simulink model "main_22a"  (R2022a)
settings: Solver=ode4  StartTime=0.0  StopTime=1  FixedStep=deltat  RelTol=1e-3
model workspace (MAT data in the model file):
  Dutyfactor = Simulink.Parameter
  Dutyfactor.Value = 0.25
  Dutyfactor.DataType = 'double'
  Dutyfactor.Complexity = 'real'
  Dutyfactor.Dimensions = [1 1]
  LenghtOfBot = Simulink.Parameter
  LenghtOfBot.Value = 0.5
  LenghtOfBot.DataType = 'double'
  LenghtOfBot.Complexity = 'real'
  LenghtOfBot.Dimensions = [1 1]
  MomentOfInertia = Simulink.Parameter
  MomentOfInertia.Value = [0.41  0  0; 0  2.1  0; 0  0  2.1]
  MomentOfInertia.DataType = 'double'
  MomentOfInertia.Complexity = 'real'
  MomentOfInertia.Dimensions = [3 3]
  Q = Simulink.Parameter
  Q.Value = [100  0  0  0  0  0  0  0  0  0  0  0; 0  100  0  0  0  0  0  0  0  0  0  0; 0  0  100  0  0  0  0  0  0  0  0  0; 0  0  0  100  0  0  0  0  0  0  0  0; 0  0  0  0  100  0  0  0  0  0  0  0; 0  0  0  0  0  100  0  0  0  0  0  0; 0  0  0  0  0  0  100  0  0  0  0  0; 0  0  0  0  0  0  0  100  0  0  0  0; 0  0  0  0  0  0  0  0  100  0  0  0; 0  0  0  0  0  0  0  0  0  100  0  0; 0  0  0  0  0  0  0  0  0  0  100  0; 0  0  0  0  0  0  0  0  0  0  0  100]
  Q.DataType = 'double'
  Q.Complexity = 'real'
  Q.Dimensions = [12 12]
  R = Simulink.Parameter
  R.Value = [1e-05  0  0  0  0  0  0  0  0  0  0  0; 0  1e-05  0  0  0  0  0  0  0  0  0  0; 0  0  1e-05  0  0  0  0  0  0  0  0  0; 0  0  0  1e-05  0  0  0  0  0  0  0  0; 0  0  0  0  1e-05  0  0  0  0  0  0  0; 0  0  0  0  0  1e-05  0  0  0  0  0  0; 0  0  0  0  0  0  1e-05  0  0  0  0  0; 0  0  0  0  0  0  0  1e-05  0  0  0  0; 0  0  0  0  0  0  0  0  1e-05  0  0  0; 0  0  0  0  0  0  0  0  0  1e-05  0  0; 0  0  0  0  0  0  0  0  0  0  1e-05  0; 0  0  0  0  0  0  0  0  0  0  0  1e-05]
  R.DataType = 'double'
  R.Complexity = 'real'
  R.Dimensions = [12 12]
  RelativePhase = Simulink.Parameter
  RelativePhase.Value = [0; 0.5; 0.75; 0.25]
  RelativePhase.DataType = 'double'
  RelativePhase.Complexity = 'real'
  RelativePhase.Dimensions = [4 1]
  WidthOfBot = Simulink.Parameter
  WidthOfBot.Value = 0.3
  WidthOfBot.DataType = 'double'
  WidthOfBot.Complexity = 'real'
  WidthOfBot.Dimensions = [1 1]
  cycleTime = Simulink.Parameter
  cycleTime.Value = 1
  cycleTime.DataType = 'double'
  cycleTime.Complexity = 'real'
  cycleTime.Dimensions = [1 1]
  deltat = Simulink.Parameter
  deltat.Value = 0.05
  deltat.DataType = 'double'
  deltat.Complexity = 'real'
  deltat.Dimensions = [1 1]
  fmax = Simulink.Parameter
  fmax.Value = 666
  fmax.DataType = 'double'
  fmax.Complexity = 'real'
  fmax.Dimensions = [1 1]
  fmin = Simulink.Parameter
  fmin.Value = 10
  fmin.DataType = 'double'
  fmin.Complexity = 'real'
  fmin.Dimensions = [1 1]
  gravity = Simulink.Parameter
  gravity.Value = [0; 0; -9.8]
  gravity.DataType = 'double'
  gravity.Complexity = 'real'
  gravity.Dimensions = [3 1]
  mass = Simulink.Parameter
  mass.Value = 43
  mass.DataType = 'double'
  mass.Complexity = 'real'
  mass.Dimensions = [1 1]
  mu = Simulink.Parameter
  mu.Value = 0.6
  mu.DataType = 'double'
  mu.Complexity = 'real'
  mu.Dimensions = [1 1]
  nominal_height = Simulink.Parameter
  nominal_height.Value = 0.2
  nominal_height.DataType = 'double'
  nominal_height.Complexity = 'real'
  nominal_height.Dimensions = [1 1]
  number_of_timeStepsMPC = Simulink.Parameter
  number_of_timeStepsMPC.Value = 1
  number_of_timeStepsMPC.DataType = 'int8'
  number_of_timeStepsMPC.Complexity = 'real'
  number_of_timeStepsMPC.Dimensions = [1 1]
values from neighbouring files (symbols this model uses):
  fmax = 660    [main24.m]
  fmin = 10    [main24.m]
  mu = 0.6    [main24.m]
  Q = zeros(13*n_steps,13*n_steps)    [Active_set_QP.m]    (also in main24.m = eye(12,12)*100)
  R = zeros(size(Bqp,2),size(Bqp,2))    [Active_set_QP.m]    (also in Aqp_Bqp.m = [0 -r(3) r(2);r(3) 0 -r(1);-r(2) r(1) 0]; main24.m = eye(12,12)*10^-2)
settings Model: Creator=user  LastModifiedBy=user
settings ModelReferenceCC: EnableRefExpFcnMdlSchedulingChecks=off
settings RTWCC: Description=Generic Real-Time Target

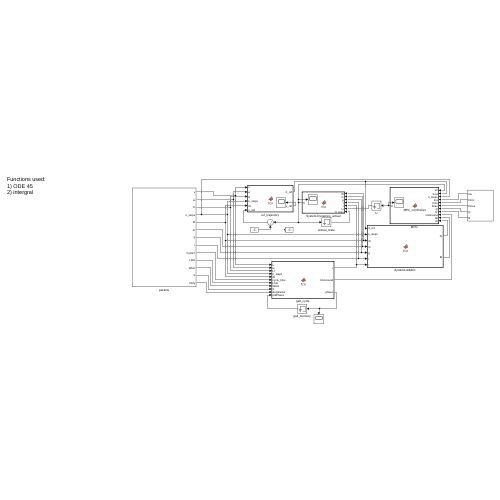
[thumbnail: Simulink's stored preview of the top-level diagram]
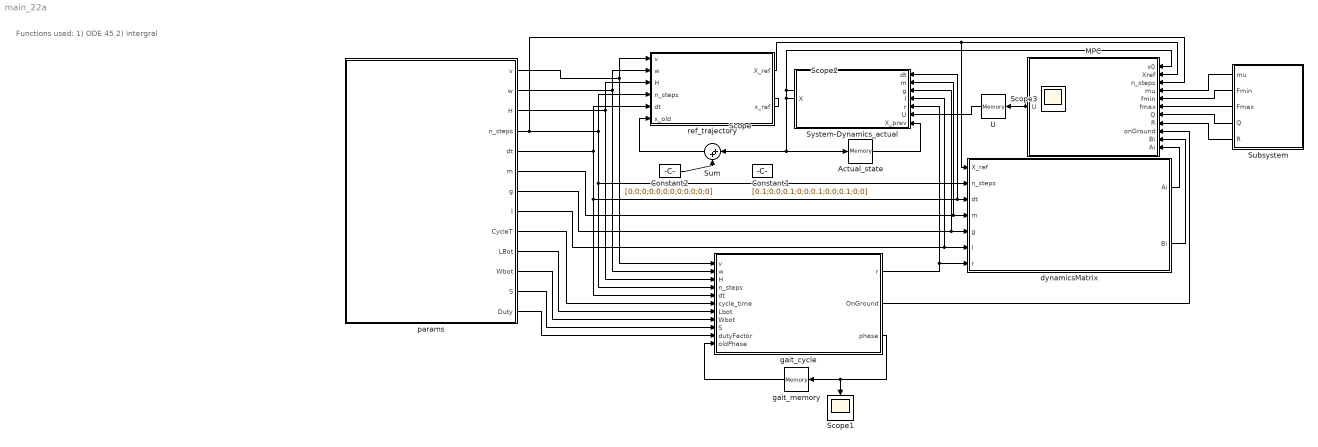
== system main_22a ==
  note: Functions used:
      | 1) ODE 45
      | 2) intergral
  Actual_state : Memory
  Constant1 : Constant  Value=[0.1;0;0;0.1;0;0;0.1;0;0;0.1;0;0]  VectorParams1D=off
  Constant2 : Constant  Value=[0;0;0;0;0;0;0;0;0;0;0;0]  VectorParams1D=off
  MPC : MATLAB Function  TreatAsAtomicUnit=on
  Scope{,1..3} (4 alike) : Scope
  Subsystem : Subsystem
  Sum : Sum  Inputs=|++
  System-Dynamics_actual : MATLAB Function  TreatAsAtomicUnit=on
  U : Memory
  dynamicsMatrix : MATLAB Function  TreatAsAtomicUnit=on
  gait_cycle : MATLAB Function  TreatAsAtomicUnit=on
  gait_memory : Memory
  params : Subsystem
  ref_trajectory : MATLAB Function  TreatAsAtomicUnit=on
  wires:
  params/1(v) -> ref_trajectory/1(v), gait_cycle/1(v)
  params/2(w) -> gait_cycle/2(w), ref_trajectory/2(w)
  params/3(H) -> gait_cycle/3(H), ref_trajectory/3(H)
  params/4(n_steps) -> MPC/3(n_steps), gait_cycle/4(n_steps), dynamicsMatrix/2(n_steps), ref_trajectory/4(n_steps)
  ref_trajectory/2(x_ref) -> Scope/1
  params/5(dt) -> gait_cycle/5(dt), dynamicsMatrix/3(dt), System-Dynamics_actual/1(dt), ref_trajectory/5(dt)
  params/9(CycleT) -> gait_cycle/6(cycle_time)
  params/10(LBot) -> gait_cycle/7(Lbot)
  params/11(Wbot) -> gait_cycle/8(Wbot)
  gait_memory/1 -> gait_cycle/11(oldPhase)
  ref_trajectory/1(X_ref) -> dynamicsMatrix/1(X_ref), MPC/2(Xref)
  params/6(m) -> dynamicsMatrix/4(m), System-Dynamics_actual/2(m)
  params/7(g) -> dynamicsMatrix/5(g), System-Dynamics_actual/3(g)
  gait_cycle/1(r) -> dynamicsMatrix/7(r), System-Dynamics_actual/5(r)
  params/12(S) -> gait_cycle/9(S)
  params/13(Duty) -> gait_cycle/10(dutyFactor)
  params/8(I) -> dynamicsMatrix/6(I), System-Dynamics_actual/4(I)
  System-Dynamics_actual/1(X) -> Actual_state/1, Sum/1, Scope2/1, MPC/1(x0)
  Actual_state/1 -> System-Dynamics_actual/7(X_prev)
  gait_cycle/3(phase) -> gait_memory/1, Scope1/1
  Sum/1 -> ref_trajectory/6(x_old)
  Constant2/1 -> Sum/2
  gait_cycle/2(OnGround) -> MPC/9(onGround)
  Subsystem/1(mu) -> MPC/4(mu)
  Subsystem/2(Fmin) -> MPC/5(fmin)
  Subsystem/3(Fmax) -> MPC/6(fmax)
  Subsystem/4(Q) -> MPC/7(Q)
  Subsystem/5(R) -> MPC/8(R)
  dynamicsMatrix/1(Ai) -> MPC/11(Ai)
  dynamicsMatrix/2(Bi) -> MPC/10(Bi)
  MPC/1(U) -> U/1, Scope3/1
  U/1 -> System-Dynamics_actual/6(U)

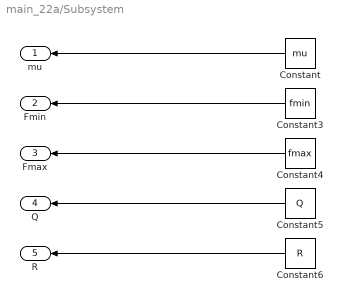
== system main_22a/Subsystem ==
  Constant : Constant  Value=mu
  Constant3 : Constant  Value=fmin
  Constant4 : Constant  Value=fmax
  Constant5 : Constant  Value=Q
  Constant6 : Constant  Value=R
  mu : Outport
  Fmin : Outport  Port=2
  Fmax : Outport  Port=3
  Q : Outport  Port=4
  R : Outport  Port=5
  wires:
  Constant3/1 -> Fmin/1
  Constant4/1 -> Fmax/1
  Constant6/1 -> R/1
  Constant5/1 -> Q/1
  Constant/1 -> mu/1

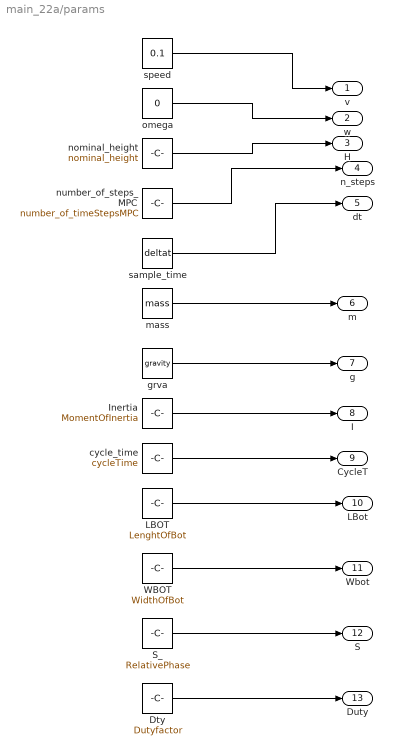
== system main_22a/params ==
  Dty : Constant  Value=Dutyfactor
  Inertia : Constant  Value=MomentOfInertia
  LBOT : Constant  Value=LenghtOfBot
  S_ : Constant  Value=RelativePhase
  WBOT : Constant  Value=WidthOfBot
  cycle_time : Constant  Value=cycleTime
  grva : Constant  Value=gravity
  mass : Constant  Value=mass
  nominal_height : Constant  Value=nominal_height
  number_of_steps_MPC : Constant  Value=number_of_timeStepsMPC
  omega : Constant  Value=0
  sample_time : Constant  Value=deltat
  speed : Constant  Value=0.1
  v : Outport
  w : Outport  Port=2
  H : Outport  Port=3
  n_steps : Outport  Port=4
  dt : Outport  Port=5
  m : Outport  Port=6
  g : Outport  Port=7
  I : Outport  Port=8
  CycleT : Outport  Port=9
  LBot : Outport  Port=10
  Wbot : Outport  Port=11
  S : Outport  Port=12
  Duty : Outport  Port=13
  wires:
  number_of_steps_MPC/1 -> n_steps/1
  omega/1 -> w/1
  nominal_height/1 -> H/1
  speed/1 -> v/1
  sample_time/1 -> dt/1
  cycle_time/1 -> CycleT/1
  LBOT/1 -> LBot/1
  WBOT/1 -> Wbot/1
  mass/1 -> m/1
  grva/1 -> g/1
  Dty/1 -> Duty/1
  S_/1 -> S/1
  Inertia/1 -> I/1

== matlab function main_22a/gait_cycle ==
  data: v input; w input; H input; n_steps input; r output size=[3,4,500]; OnGround output size=[4,500]; dt input; cycle_time input; Lbot input; Wbot input; S input; dutyFactor input; oldPhase input; phase output double size=1
function [r,OnGround,phase] = fcn(v,w,H,n_steps,dt,cycle_time,Lbot,Wbot,S,dutyFactor,oldPhase)
    vr=(2*v+w*Wbot)/2;
    vl=(2*v-w*Wbot)/2;
    LstanceR=cycle_time*(1-dutyFactor)*vl;
    LstanceL=cycle_time*(1-dutyFactor)*vr;
    OnGround=zeros(4,n_steps);
    r=zeros(3,4,n_steps);
    phase=oldPhase;
    for k=1:n_steps
        phase=mod(phase+dt/cycle_time,1);
        for i=1:4           
            phase_leg=mod(phase+S(i),1);
            if(phase_leg>dutyFactor)
                OnGround(i,k)=1;
                if(i==1 || i==3)                 
                    r(:,i,k)=[LstanceL*(phase_leg/dutyFactor -0.5);0;0];             
                else
                    r(:,i,k)=[LstanceR*(phase_leg/dutyFactor -0.5);0;0];
                end                
            else
                r(:,i,k)=[0;0;H*0.25];
            end
        end
        r(:,:,k)=r(:,:,k)+[[Lbot/2;Wbot/2;-H],[Lbot/2;-Wbot/2;-H],[-Lbot/2;Wbot/2;-H],[-Lbot/2;-Wbot/2;-H]];
    end
    phase=mod(oldPhase+dt/cycle_time,1);
end

== matlab function main_22a/ref_trajectory ==
  settings: updateMethod=DISCRETE  sampleTime=deltat
  data: v input; X_ref output double size=[12,500]; w input; H input; n_steps input; dt input; x_old input; x_ref output double size=[12 1]
function [X_ref,x_ref] = fcn(v,w,H,n_steps, dt,x_old)
    X_ref=zeros(12,n_steps);
    X_ref(4,1)=x_old(4,1);
    X_ref(5,1)=x_old(5,1);
    X_ref(3,1)=x_old(3,1);
    for i=0:(n_steps-1)
        X_ref(4,i+1)=X_ref(4,i+1)+v*dt*cos(X_ref(3,i+1));
        X_ref(5,i+1)=X_ref(5,i+1)+v*dt*sin(X_ref(3,i+1));
        X_ref(6,i+1)=0;        
        X_ref(10,i+1)=v*cos(X_ref(3,i+1));
        X_ref(11,i+1)=v*sin(X_ref(3,i+1));
        X_ref(3,i+1)=X_ref(3,i+1)+w*dt;
        X_ref(9,i+1)=w;
        if(i<(n_steps-1))
            X_ref(:,i+2)=X_ref(:,i+1);
        end
    end
    x_ref=X_ref(:,1);
    % ground Air
    %Ri
end

== matlab function main_22a/dynamicsMatrix ==
  data: X_ref input; n_steps input; dt input; Ai output double size=[12,12,500]; m input; g input; I input; r input; Bi output double size=[12,13,500]
function [Ai,Bi] = fcn(X_ref,n_steps,dt,m,g,I,r)
    Ai=zeros(12,12,n_steps);
    Bi=zeros(12,13,n_steps);
    for k=1:n_steps
        R=[cos(X_ref(3,k)), sin(X_ref(3,k)), 0;
          -sin(X_ref(3,k)), cos(X_ref(3,k)), 0;
                         0,               0, 1];
       I_=(R*I*R')^-1;
                
        A=[zeros(3), zeros(3),        R, zeros(3);
           zeros(3), zeros(3), zeros(3),   eye(3);
           zeros(3), zeros(3), zeros(3), zeros(3);
           zeros(3), zeros(3), zeros(3), zeros(3);];
        
        B=[      zeros(3),        zeros(3),        zeros(3),        zeros(3), zeros(3,1);
                 zeros(3),        zeros(3),        zeros(3),        zeros(3), zeros(3,1);
          I_*CP(r(:,1,1)), I_*CP(r(:,2,1)), I_*CP(r(:,3,1)), I_*CP(r(:,4,1)), zeros(3,1);
                eye(3)./m,       eye(3)./m,       eye(3)./m,       eye(3)./m,         g];
       
       Ai(:,:,k)=exp(A.*dt);
       Bi(:,:,k)=integral(@(t) exp(A.*t)*B,0,dt,"ArrayValued",true);

    end

    function R = CP(r)
        R=[0 -r(3) r(2);r(3) 0 -r(1);-r(2) r(1) 0];
    end
end

== matlab function main_22a/System-Dynamics_actual ==
  data: dt input; X output size=[12 1]; m input; g input; I input; r input; U input; X_prev input
function X  = fcn(dt,m,g,I,r,U,X_prev)     
    [t,y] = ode45(@dynamics_eq ,[0 dt],X_prev);
    X=y(end,:)';
    function dxdt=dynamics_eq(t,y)
        R=[cos(y(3)), sin(y(3)), 0;
         - sin(y(3)), cos(y(3)), 0;
                   0,         0, 1];
        I_=(R*I*R')^-1;        
        A=[zeros(3), zeros(3),        R, zeros(3);
           zeros(3), zeros(3), zeros(3),  eye(3);
           zeros(3), zeros(3), zeros(3), zeros(3);
           zeros(3), zeros(3), zeros(3), zeros(3);];
        
        B=[      zeros(3),        zeros(3),        zeros(3),        zeros(3), zeros(3,1);
                 zeros(3),        zeros(3),        zeros(3),        zeros(3), zeros(3,1);
          I_*CP(r(:,1,1)), I_*CP(r(:,2,1)), I_*CP(r(:,3,1)), I_*CP(r(:,4,1)), zeros(3,1);
                eye(3)./m,       eye(3)./m,       eye(3)./m,       eye(3)./m,         g];
        dxdt=A*y+B*[U;1];
    end

    function R = CP(r)
        R=[0 -r(3) r(2);r(3) 0 -r(1);-r(2) r(1) 0];
    end
end

== matlab function main_22a/MPC ==
  data: x0 input; Xref input; n_steps input; mu input; fmin input; fmax input; Q input; R input; onGround input; Bi input; Ai input; U output size=[12 1]
function U  = MPC_controller(x0,Xref,n_steps,mu,fmin,fmax,Q,R,onGround,Bi,Ai)
    coder.extrinsic('Active_set');
    out=Active_set(x0,Xref,n_steps,mu,fmin,fmax,Q,R,onGround,Bi,Ai);
    U=zeros(12,1);
    U(:,1)=out;
end
